simulink model "MtrCtrl_24V"  (R2023b)
settings: Solver=FixedStepDiscrete  StartTime=0.0  StopTime=1  FixedStep=1e-6  RelTol=1e-3
values from neighbouring files (symbols this model uses):
  B = 0.001889    [MtrCtrl_v01.sldd]    (also in PICal.m = 0.001889; PMSM.m = Simulink.Parameter)
  C_LUT_AngleTable_sng_Null = saveVarsMat.C_LUT_AngleTable_sng_Null    [AngleTable.m]    (also in MtrCtrl_v01.sldd = 0.0015339807878856412 0.0030679615757712823 0.00460194236365; PMSM.m; SinLut.m = sinTable(2,:))
  C_LUT_SinTable_sng_Null = saveVarsMat.C_LUT_SinTable_sng_Null    [AngleTable.m]    (also in MtrCtrl_v01.sldd = 0.0015339801862847655 0.0030679567629659761 0.00460192612044; PMSM.m; SinLut.m = sinTable(1,:))
  C_MATH_OneOverSqrtThree_s32n31_Null = 0.57735026918962584    [MtrCtrl_v01.sldd]    (also in PMSM.m = Simulink.Parameter)
  C_MATH_Pi_u32n30_Null = 3.1415926535897931    [MtrCtrl_v01.sldd]    (also in PMSM.m = Simulink.Parameter)
  C_MATH_SqrtThreeOverThree_s32n31_Null = 0.57735026918962573    [MtrCtrl_v01.sldd]    (also in PMSM.m = Simulink.Parameter)
  C_PMSM_CurQKi_u32n31_null = 0.15707963267949    [MtrCtrl_v01.sldd]    (also in PMSM.m = Simulink.Parameter)
  C_PMSM_CurQKp_u32n31_null = 19.949113350295185    [MtrCtrl_v01.sldd]    (also in PMSM.m = Simulink.Parameter)
  C_PMSM_Flux_u32n32_Vs = 0.192    [MtrCtrl_v01.sldd]    (also in PMSM.m = Simulink.Parameter)
  C_PMSM_Ls_pu = 0.398982267005904    [MtrCtrl_v01.sldd]
  C_PMSM_PolePairs_u8_Null = 4.0    [MtrCtrl_v01.sldd]
  Flux = 0.192    [MtrCtrl_v01.sldd]    (also in PICal.m; PMSM.m)
  IBase_A = 2000.0    [MtrCtrl_v01.sldd]    (also in PICal.m = 300; PMSM.m = Simulink.Parameter)
  J = 0.011    [MtrCtrl_v01.sldd]    (also in PICal.m; PMSM.m)
  K_CCM_MRASEna_bool_Flg = 0.0    [MtrCtrl_v01.sldd]
  K_SVM_DefultDuty_s32n31_Null = 0.25    [MtrCtrl_v01.sldd]    (also in PMSM.m = Simulink.Parameter)
  KCCM_VirPosn_flg = 0.0    [MtrCtrl_v01.sldd]    (also in PMSM.m = Simulink.Parameter)
  KCCM_VoltModeEna_Flg = 0.0    [MtrCtrl_v01.sldd]    (also in PMSM.m = Simulink.Parameter)
  Kis = 114583.3333333333    [MtrCtrl_v01.sldd]    (also in PICal.m = 114583.333333; PMSM.m = 114583.333333)
  KSMO_EnaEst_Flg = 0.0    [MtrCtrl_v01.sldd]    (also in PMSM.m = Simulink.Parameter)
  Kt = 1.1520000000000001    [MtrCtrl_v01.sldd]    (also in PICal.m = 1.152; PMSM.m = 1.152)
  Ld = 80e-6    (= 8e-05)    [FluxweakingGen.m]    (also in IEHB_MAPGenerationtest.m = 6.8e-05; MtrCtrl_v01.sldd = 0.000635
                
                    
             ; PICal.m = 0.000635; PMSM.m = Simulink.Parameter)
  LPF_coefg = 0.01    [MtrCtrl_v01.sldd]    (also in PMSM.m = Simulink.Parameter)
  Lq = 80e-6    (= 8e-05)    [FluxweakingGen.m]    (also in IEHB_MAPGenerationtest.m = 6e-05; MtrCtrl_v01.sldd = 0.000685
                
                    
             ; PICal.m = 0.000635; PMSM.m = Simulink.Parameter)
  Ls = 0.000635    [MtrCtrl_v01.sldd]    (also in PICal.m; PMSM.m)
  OneOverUBase_V = 0.0016666666666666668    [MtrCtrl_v01.sldd]    (also in PMSM.m = Simulink.Parameter)
  Pp = 4.0    [MtrCtrl_v01.sldd]    (also in PICal.m = 4; PMSM.m = Simulink.Parameter)
  Rs = 0.03    [FluxweakingGen.m]    (also in MtrCtrl_v01.sldd = 0.05
                
                    
                 ; PICal.m = 0.05; PMSM.m = Simulink.Parameter)
  SecPerRnd = 0.6    [MtrCtrl_v01.sldd]    (also in PMSM.m = Simulink.Parameter)
  sinTable = zeros(2,TableSize)    [SinLut.m]
  SMOGain_V = 323.31615074619043    [MtrCtrl_v01.sldd]    (also in PMSM.m = Simulink.Parameter)
  Ts = 1.0E-6    [MtrCtrl_v01.sldd]    (also in PICal.m = 0.0001; PMSM.m = Simulink.Parameter)
  TsCtrl = 1.0E-6    [MtrCtrl_v01.sldd]
  UBase_V = 600.0    [MtrCtrl_v01.sldd]    (also in PICal.m = 600; PMSM.m = Simulink.Parameter)
  wmBase_rps = 314.15926535897933    [MtrCtrl_v01.sldd]    (also in PICal.m = 314.159265359; PMSM.m = Simulink.Parameter)
undefined symbols (not defined in the file or in its folder): DiscIntNeverNeededParam, Ion, Lithium
libraries: ee_lib x16, spsVoltageMeasurementLib x14, simulink x11, spsSeriesRLCBranchLib x6, spsMosfetLib x6, nesl_utility x6, slpidlib x5, spsCurrentMeasurementLib x4, spsParallelRLCBranchLib x3, simulink_extras x2, spspowerguiLib x2, eePmsmFwController x1
(part 1 of 5)
settings Model: DataDictionary=MtrCtrl_v01.sldd  FPTShortcutValueString='{{},{''BaselineRun'',1,1,1,''BaselineRun'','''',{},''M'','''',''''}}'  PauseTimes=0.0842  NumberOfSteps=100  SnapshotBufferSize=1000  SnapshotInterval=1  Creator=ZhangZhehu  LastModifiedBy=z1486
settings OptimizationCC: DefaultParameterBehavior=Inlined  UseDivisionForNetSlopeComputation=on  GainParamInheritBuiltInType=on  UseFloatMulNetSlope=on  DefaultUnderspecifiedDataType=single  InlineInvariantSignals=on  PassReuseOutputArgsAs=Individual arguments  ZeroExternalMemoryAtStartup=off  ZeroInternalMemoryAtStartup=off  NoFixptDivByZeroProtection=on  EfficientFloat2IntCast=on  LifeSpan=1  OptimizeBlockOrder=speed  DifferentSizesBufferReuse=on  EfficientTunableParamExpr=on
settings DebuggingCC: SignalRangeChecking=warning  ParameterTunabilityLossMsg=error  UnconnectedInputMsg=warning  UnconnectedOutputMsg=warning  UnconnectedLineMsg=warning
settings HardwareCC: ProdBitPerPointer=32  ProdBitPerSizeT=32  ProdBitPerPtrDiffT=32  ProdLargestAtomicFloat=None  ProdWordSize=32  ProdLongLongMode=on  ProdHWDeviceType=Infineon->TriCore
settings ModelReferenceCC: EnableRefExpFcnMdlSchedulingChecks=on
settings SFSimCC: MATLABDynamicMemAlloc=off
settings RTWCC: Description=Embedded Coder  SystemTargetFile=ert.tlc  GenCodeOnly=on  TemplateMakefile=ert_default_tmf  BuildConfiguration=Faster Runs  DLArmComputeVersion=19.05
settings CodeAppCC: ForceParamTrailComments=on  IgnoreCustomStorageClasses=off  OperatorAnnotations=on  SimulinkDataObjDesc=on  SFDataObjDesc=on  CustomSymbolStrGlobalVar=rt$N$M  CustomSymbolStrType=$N$M  CustomSymbolStrFcn=$N$M$F  CustomSymbolStrMacro=$N$M  InsertBlockDesc=on
settings ERTTargetCC: TargetLangStandard=C99 (ISO)  GenerateSampleERTMain=on  IncludeMdlTerminateFcn=off  CombineSignalStateStructs=on  SupportComplex=off  SupportNonInlinedSFcns=on  InlinedParameterPlacement=NonHierarchical  ERTCustomFileTemplate=example_file_process.tlc  ERTFilePackagingFormat=CompactWithDataFile

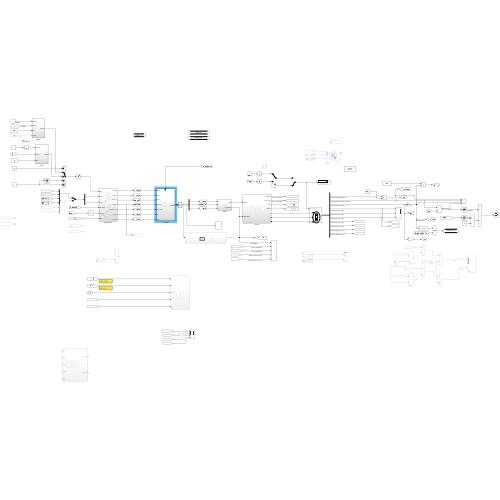
[thumbnail: Simulink's stored preview of the top-level diagram]
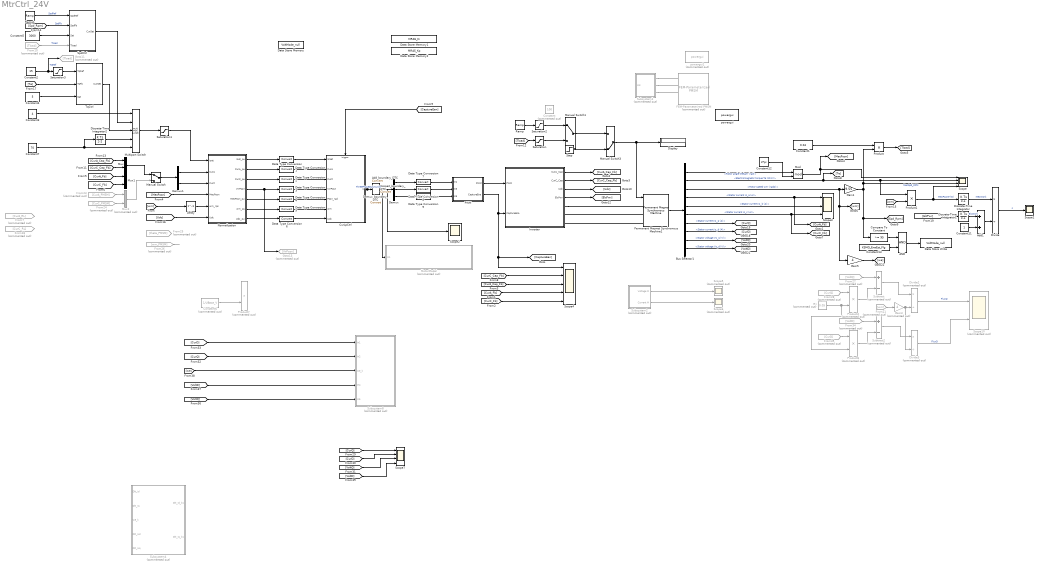
== system MtrCtrl_24V ==
  AND : Logic  AllPortsSameDT=off  OutDataTypeStr=boolean
  Add1 : Sum
  Add_boundary_DTC : DataTypeConversion
  Bus Selector1 : BusSelector  OutputSignals=Rotor angle thetam (rad),Electromagnetic torque Te (N*m),Rotor speed wm (rad/s),Stator current is_a (A),Stator current is_b (A),Stator current is_c (A),Stator current is_q (A),Stator current is_d (A),Stator voltage Vs_q (V),Stator voltage Vs_d (V)
  Compare To Constant : simulink/Logic and Bit Operations/Compare To Constant  relop=>=  const=95  OutDataTypeStr=boolean
  Constant : Constant  Commented=on  Value=100
  Constant1 : Constant  Value=0.04
  Constant11 : Constant
  Constant12 : Constant  Value=2*pi
  Constant13 : Constant  Value=KSMO_EnaEst_Flg
  Constant2 : Constant  Value=15
  Constant3 : Constant  Value=4
  Constant4 : Constant  Value=5
  Constant5 : Constant  Value=3000
  Constant6 : Constant  Commented=on  Value=1/UBase_V
  Constant7 : Constant  Value=70
  CurLpCtrl : Subsystem
      settings: RTWSystemCode=Nonreusable function  RTWFcnNameOpts=Use subsystem name
  Data Store Memory : DataStoreMemory  DataStoreName=VoltMode_null  WriteAfterWriteMsg=warning  ShowAdditionalParam=off
  Data Store Memory1 : DataStoreMemory  DataStoreName=MRAS_Ki  WriteAfterWriteMsg=warning  ShowAdditionalParam=off
  Data Store Memory2 : DataStoreMemory  DataStoreName=MRAS_Kp  WriteAfterWriteMsg=warning  ShowAdditionalParam=off  OutDataTypeStr=fixdt(1,32,27)
  Data Store Write : DataStoreWrite  DataStoreName=VoltMode_null  IndexOptions=Index vector (dialog)  Indices=1  OutputSizes=1
  Data Type Conversion{,1..9} (10 alike) : DataTypeConversion  SaturateOnIntegerOverflow=off  RndMeth=Floor
  Delay : Delay  DelayLength=1
  Demux : Demux  Outputs=3
  Demux1 : Demux  Outputs=2
  Demux_boundary_DTC : DataTypeConversion
  Discrete-Time Integrator : DiscreteIntegrator  SampleTime=-1  ICPrevOutput=DiscIntNeverNeededParam  ICPrevScaledInput=DiscIntNeverNeededParam
  Discrete-Time Integrator1 : DiscreteIntegrator  SampleTime=-1  ICPrevOutput=DiscIntNeverNeededParam  ICPrevScaledInput=DiscIntNeverNeededParam
  Discrete-Time Integrator2 : DiscreteIntegrator  SampleTime=-1  ICPrevOutput=DiscIntNeverNeededParam  ICPrevScaledInput=DiscIntNeverNeededParam
  Display : Display
  Divide : Product  Inputs=*/
  Divide2 : Product  Commented=on  Inputs=*/
  Divide3 : Product  Commented=on  Inputs=*/
  FEM-Parameterized PMSM : ee_lib/Electromechanical/Permanent Magnet/FEM-Parameterized PMSM  Commented=on  parameterization=1  winding_type=ee.enum.statorconnection.wye  iVec=[-2, 0, 2] A  xVec=[0, 20, 40, 60] deg  dfluxdiMatrix=0.0002 * ones(3, 4) Wb/A  dfluxdxMatrix=[0, -.16, .16, 0; 0, -.16, .16, 0; 0, -.16, .16, 0] Wb/rad  calculate_torque_matrix=1  TorqueMatrix=zeros(3, 3, 3, 4) N*m  idVec1=[-200, 0, 200] A  iqVec1=[-200, 0, 200] A  LdMatrix=0.0002 * ones(3, 3) H  LqMatrix=0.0002 * ones(3, 3) H  PmMatrix=0.1 * ones(3, 3) Wb  N=4  interp_method=simscape.enum.interpolation.linear  Rs=0.05 Ohm  Ms=0.00002 H  L0=0.00016 H  loss_param=ee.enum.fem_motor.ironLosses.empirical  losses_oc=[0, 0, 0] W  losses_sc=[0, 0, 0] W  f_losses=60 Hz  Isc_losses=95 A  Inertia=0.01 kg*m^2  lam=0 N*m*s/rad  i_d_specify=off  i_d_priority=None  i_d=0 A  i_d_nominal_specify=off  i_d_nominal_unit=A  i_d_nominal_value=1  i_q_specify=off  i_q_priority=None  i_q=0 A  i_q_nominal_specify=off  i_q_nominal_unit=A  i_q_nominal_value=1  torque_specify=off  torque_priority=None  torque=0 N*m  torque_nominal_specify=off  torque_nominal_unit=N*m  torque_nominal_value=1  angular_velocity_specify=off  angular_velocity_priority=High  angular_velocity=0 rpm  angular_velocity_nominal_specify=off  angular_velocity_nominal_unit=rpm  angular_velocity_nominal_value=1  angular_position_specify=off  angular_position_priority=High  angular_position=0 deg  angular_position_nominal_specify=off  angular_position_nominal_unit=deg  angular_position_nominal_value=1  Tmeas=298.15 K  alpha=3.93e-3 1/K  alpha_flux=-0.001 1/K  stator_thermal_mass=100 J/K  stator_initial_temperatures=[298.15, 298.15, 298.15] K  rotor_thermal_mass=200 J/K  rotor_initial_temperature=298.15 K  Rm_percent_rotor=90  Rd_percent_rotor=30  idVec=[-200, 0, 200] A  iqVec=[-200, 0, 200] A  dfluxAdiaMatrix3D=zeros(3, 3, 4) Wb/A  dfluxAdibMatrix3D=zeros(3, 3, 4) Wb/A  dfluxAdicMatrix3D=zeros(3, 3, 4) Wb/A  dfluxAdxMatrix3D=zeros(3, 3, 4) Wb/rad  TorqueMatrix3D=zeros(3, 3, 4) N*m  iaVec=[-200, 0, 200] A  ibVec=[-200, 0, 200] A  icVec=[-200, 0, 200] A  dfluxAdiaMatrix=zeros(3, 3, 3, 4) Wb/A  dfluxAdibMatrix=zeros(3, 3, 3, 4) Wb/A  dfluxAdicMatrix=zeros(3, 3, 3, 4) Wb/A  dfluxAdxMatrix=zeros(3, 3, 3, 4) Wb/rad  param_dq0=ee.enum.fem_motor.fluxTabulationOption.DQcartesian  winding_type_dq0=ee.enum.statorconnection.wye  expose_neutral_port=ee.enum.fem_motor.exposeNeutralPort.no  nPolePairs=4  parks_type=ee.enum.fem_motor.parksType.QleadsD_AphaseToDaxis  idVec2=[-200, 0, 200] A  iqVec2=[-200, 0, 200] A  magVec2=[0, 100, 200] A  betaVec2=[-180, -90, 0, 90, 180] deg  xVec2=[0, 15, 30, 45, 60, 75, 90] deg  fluxD_dq0=zeros(3, 3, 7) Wb  fluxQ_dq0=zeros(3, 3, 7) Wb  fluxA_dq0=zeros(3, 3, 7) Wb  Torque_dq0=ones(3, 3, 7) N*m  fluxD_IBX=zeros(3, 5, 7) Wb  fluxQ_IBX=zeros(3, 5, 7) Wb  fluxA_IBX=zeros(3, 5, 7) Wb  Torque_IBX=zeros(3, 5, 7) N*m  rotorLossCoeff_k_h_DQ=zeros(3, 3) W/Hz  rotorLossCoeff_k_J_DQ=zeros(3, 3) W/Hz^2  rotorLossCoeff_k_ex_DQ=zeros(3, 3) W/Hz^(3/2)  rotorLossCoeff_k_h_IB=zeros(3, 5) W/Hz  rotorLossCoeff_k_J_IB=zeros(3, 5) W/Hz^2  rotorLossCoeff_k_ex_IB=zeros(3, 5) W/Hz^(3/2)  statorLossCoeff_k_h_DQ=zeros(3, 3) W/Hz  statorLossCoeff_k_J_DQ=zeros(3, 3) W/Hz^2  statorLossCoeff_k_ex_DQ=zeros(3, 3) W/Hz^(3/2)  statorLossCoeff_k_h_IB=zeros(3, 5) W/Hz  statorLossCoeff_k_J_IB=zeros(3, 5) W/Hz^2  statorLossCoeff_k_ex_IB=zeros(3, 5) W/Hz^(3/2)  wVec=[1000, 2000] rpm  rotorLossTable_DQ=zeros(3, 3, 2) W  rotorLossTable_IB=zeros(3, 5, 2) W  statorLossTable_DQ=zeros(3, 3, 2) W  statorLossTable_IB=zeros(3, 5, 2) W  electrical_torque_before_iron_losses_specify=off  electrical_torque_before_iron_losses_priority=None  electrical_torque_before_iron_losses=0 N*m  electrical_torque_before_iron_losses_nominal_specify=off  electrical_torque_before_iron_losses_nominal_unit=N*m  electrical_torque_before_iron_losses_nominal_value=1  Qrotor_specify=off  Qrotor_priority=None  Qrotor=0 J/s  Qrotor_nominal_specify=off  Qrotor_nominal_unit=J/s  Qrotor_nominal_value=1  Qstator_specify=off  Qstator_priority=None  Qstator=0 J/s  Qstator_nominal_specify=off  Qstator_nominal_unit=J/s  Qstator_nominal_value=1
      settings: InternalSimscapePortConfiguration="{\"Bottom\":[],\"Left\":[{\"id\":\"a\",\"label\":\"a\",\"type\":\"foundation.electrical.electrical\"},{\"id\":\"b\",\"label\":\"b\",\"type\":\"foundation.electrical.electrical\"},{\"id\":\"c\",\"label\":\"c\",\"type\":\"foundation.electrical.electrical\"},{\"id\":\"n\",\"label\":\"n\",\"type\":\"foundation.electrical.electrical\"}],\"Right\":[{\"id\":\"R\",\"label\":\"R\",\"type\":\"foundation.mechanical.rotational.rotational\"},{\"id\":\"C\",\"label\":\"C\",\"type\":\"foundation.mechanical.rotational.rotational\"}],\"Top\":[]}"
  From10 : From  Commented=on  GotoTag=Tload
  From18 : From  Commented=on  GotoTag=CurC_RL
  From21 : From  Commented=on  GotoTag=wm
  From23 : From  Commented=on  GotoTag=CurA_PMSM
  From24 : From  Commented=on  GotoTag=CurC_PMSM
  From25 : From  Commented=on  GotoTag=theta_PMSM
  From26 : From  Commented=on  GotoTag=wm_PMSM
  From27 : From  Commented=on  GotoTag=VoltQ
  From28 : From  Commented=on  GotoTag=CurQ
  From34 : From  Commented=on  GotoTag=VoltD
  From35 : From  Commented=on  GotoTag=CurD
  From7 : From  Commented=on  GotoTag=CurA_RL
  Gain1 : Gain  Gain=9.55
  Gain3 : Gain  Commented=on  Gain=4
  Gain5 : Gain  Gain=4
  Goto11 : Goto  Commented=on  GotoTag=Tload
  Goto13 : Goto  Commented=on  GotoTag=VirPosn
  Inverter : Subsystem
  Manual Switch : ManualSwitch
  Manual Switch1 : ManualSwitch
  Manual Switch3 : ManualSwitch  CurrentSetting=0
  Mod : Math  Operator=mod
  MotorModel : Subsystem  Commented=on
  Multiport Switch : MultiPortSwitch  Inputs=4  SaturateOnIntegerOverflow=off  InputSameDT=off
  Mux : Mux  Inputs=2
  Mux1 : Mux  Inputs=2
  Mux2 : Mux  Commented=on  Inputs=2
  Normalization : Subsystem
  PWM : Subsystem
  Permanent Magnet Synchronous Machine1 : spsPermanentMagnetSynchronousMachineLib/Permanent Magnet Synchronous Machine  NbPhases=3  FluxDistribution=Sinusoidal  RotorType=Round  MechanicalLoad=Speed w  PresetModel=No  ShowDetailedParameters=on  MeasurementBus=off  Resistance=0.05  Inductance=6.5e-5  dqInductances=[8.5e-3,8.5e-3]  La=0.000635  MachineConstant=Flux linkage established by magnets (V.s)  Flux=0.192  VoltageCst=139.2998  TorqueCst=1.152  Flat=120  Mechanical=[0.011 0.001889 4 0]  PolePairs=4  InitialConditions=[0,0, 0,0]  InitialConditions5ph=[0 0 0 0 0 0]  RefAngle=Aligned with phase A axis (original Park)  IterativeDiscreteModel=Trapezoidal non iterative  TsBlock=-1  TsPowergui=0
  Product : Product
  Product1 : Product
  Product2 : Product  Commented=on
  Product4 : Product  Commented=on
  Product8 : Product  Commented=on
  Ramp : simulink/Sources/Ramp  slope=30  start=0  InitialOutput=0
  Ramp1 : simulink/Sources/Ramp  slope=2000  start=0  InitialOutput=0
  Rs : Constant  Commented=on  Value=0.05
  Saturation : Saturate  UpperLimit=200  LowerLimit=-5
  Saturation1 : Saturate  UpperLimit=220
  Saturation2 : Saturate  UpperLimit=30
  Saturation3 : Saturate  UpperLimit=11
  Scope : Scope  NumInputPorts=4
  Scope1 : Scope
  Scope10 : Scope  Commented=on  NumInputPorts=2
  Scope2 : Scope
  Scope2_boundary_DTC : DataTypeConversion
  Scope3 : Scope  NumInputPorts=3
  Scope4 : Scope  NumInputPorts=5
  Scope5 : Scope  Commented=on
  Scope6 : Scope  Commented=on
  Scope7 : Scope  NumInputPorts=4
  SpdCtrl : Subsystem
  Step : Step  Time=0.01  After=100  SampleTime=0
  Subsystem1 : Subsystem  Commented=on
  Subsystem2 : Subsystem  Commented=on
  Subsystem4 : Subsystem  Commented=on
  Subsystem8 : Subsystem  Commented=on
  Subtract : Sum  Commented=on  Inputs=+-
  Subtract2 : Sum  Commented=on  Inputs=+-
  TqCtrl : Subsystem
  powergui : spspowerguiLib/powergui  Priority=1  SimulationMode=Discrete  SampleTime=1e-6  frequency=60  Iterations=50  frequencyindice=0  Pbase=100e6  ErrMax=1e-4  UnitsV=kV  UnitsW=MW  buscounter=0  FunctionMessages=off  echomessages=off  EnableUseOfTLC=off  CurrentSourceSwitches=off  DisableSnubberDevices=off  DisableRonSwitches=off  DisableVfSwitches=off  DisplayEquations=off  AutomaticDiscreteSolvers=off  SolverType=Tustin/Backward Euler (TBE)  Interpol=off  ExternalGateDelay=off  methode=off  Ts=100  x0status=blocks  SPID=on  SwTol=0  HookPort=off  NonlinearTolerance=1e-4  nMaxIteration=100  ContinueOnMaxIteration=off  RestoreLinks=warning  ResistiveCurrentMeasurement=off  Frange=[0:2:500]  Ylog=off  Xlog=on  ShowGrid=off  save=off  variable=ZData  structure=0  ZoomFFT=off  StartTime=0.0  cycles=1  DisplayStyle=1  fundamental=60  FreqAxis=off  MaxFrequency=1000  frequencyindicesteady=1  RmsSteady=1  display=off
  powergui1 : spspowerguiLib/powergui  Priority=1  Commented=on  SimulationMode=Continuous  SampleTime=50e-6  frequency=60  Iterations=50  frequencyindice=60  Pbase=100e6  ErrMax=1e-4  UnitsV=kV  UnitsW=MW  buscounter=0  FunctionMessages=off  echomessages=off  EnableUseOfTLC=off  CurrentSourceSwitches=off  DisableSnubberDevices=off  DisableRonSwitches=off  DisableVfSwitches=off  DisplayEquations=off  AutomaticDiscreteSolvers=off  SolverType=Tustin/Backward Euler (TBE)  Interpol=off  ExternalGateDelay=off  methode=off  Ts=100  x0status=blocks  SPID=on  SwTol=0  HookPort=off  NonlinearTolerance=1e-4  nMaxIteration=100  ContinueOnMaxIteration=off  RestoreLinks=warning  ResistiveCurrentMeasurement=off  Frange=[0:2:500]  Ylog=off  Xlog=on  ShowGrid=off  save=off  variable=ZData  structure=0  ZoomFFT=off  StartTime=0.0  cycles=1  DisplayStyle=1  fundamental=60  FreqAxis=off  MaxFrequency=1000  frequencyindicesteady=1  RmsSteady=1  display=off
  wires:
  Ramp/1 -> Saturation2/1
  Bus Selector1/4 -> Scope3/1, [CurA_Fb]  "<Stator current is_a (A)>"
  Bus Selector1/2 -> [Te], Scope/2, Product1/1  "<Electromagnetic torque Te (N*m)>"
  Mod/1 -> [MecPosn], Scope/1
  Permanent Magnet Synchronous Machine1/1 -> Bus Selector1/1
  Bus Selector1/6 -> Scope3/3, [CurC_Fb]  "<Stator current is_c (A)>"
  Bus Selector1/3 -> Gain5/1, [wm], Gain1/1  "<Rotor speed wm (rad/s)>"
  Gain1/1 -> Compare To Constant/1, [Spd_Rpm], Product/2, Scope/3  "MecSpd_RPM"
  Constant1/1 -> Product/1
  Product/1 -> [Tload]
  PWM/1(PWM) -> Inverter/1(PWM)
  Demux/3 -> Data Type Conversion9/1
  Demux/1 -> Data Type Conversion7/1
  Demux/2 -> Data Type Conversion8/1
  PWM/2(CaptureEna) -> [CaptureEan], Scope4/1, Inverter/2(CaptureEna)
  From26/1 -> ?
  Inverter/2(CurC_Cap) -> [CurC_Cap_Fb]
  Inverter/1(CurA_Cap) -> [CurA_Cap_Fb]
  Bus Selector1/5 -> Scope3/2  "<Stator current is_b (A)>"
  [CurA_Fb] -> Scope4/4
  [CurC_Fb] -> Scope4/5
  [CurC_Cap_Fb] -> Scope4/2
  [CurA_Cap_Fb] -> Scope4/3
  [CaptureEan] -> CurLpCtrl/Trigger
  [wm] -> Product1/2
  Inverter/3(Udc) -> [Udc]
  Ramp1/1 -> SpdCtrl/1(SpdRef)  "SpdRef"
  [Spd_Rpm] -> SpdCtrl/2(SpdFb)  "SpdFb"
  Constant5/1 -> SpdCtrl/3(Sat)
  From10/1 -> SpdCtrl/4(Tload)  "Tload"
  SpdCtrl/1(CurSet) -> Multiport Switch/2
  TqCtrl/1(CurSet) -> Multiport Switch/3
  [Te] -> TqCtrl/2(TqFb)
  Constant2/1 -> Goto11/1, Saturation3/1  "TqRef"
  Constant4/1 -> TqCtrl/3(Sat)
  [Tload] -> Saturation/1
  Saturation/1 -> Manual Switch1/2
  Saturation2/1 -> Manual Switch1/1
  Manual Switch/1 -> Demux1/1
  Mux2/1 -> Manual Switch/2
  [CurC_Cap_Fb] -> Mux/2
  [CurA_Cap_Fb] -> Mux/1
  Mux/1 -> Manual Switch/1
  [CurC_Fb] -> Mux1/2
  [CurA_Fb] -> Mux1/1
  Manual Switch3/1 -> Display/1, Permanent Magnet Synchronous Machine1/1
  Manual Switch1/1 -> Manual Switch3/1
  Product1/1 -> Discrete-Time Integrator/1, Scope/4  "MecPower(W)"
  Saturation3/1 -> TqCtrl/1(TqRef)
  Inverter/4(ElcPwr) -> [ElcPwr]
  Discrete-Time Integrator/1 -> Divide/1  "MecWork"
  [ElcPwr] -> Discrete-Time Integrator1/1
  Discrete-Time Integrator1/1 -> Add1/1  "ElcWork"
  Divide/1 -> Scope1/1  "n"
  Step/1 -> Manual Switch3/2
  Constant6/1 -> Product2/2
  Multiport Switch/1 -> Saturation1/1
  Demux1/1 -> Normalization/2(CurA)
  Demux1/2 -> Normalization/3(CurC)
  [MecPosn] -> Normalization/4(MecPosn)
  Delay/1 -> Normalization/5(wm_rps)
  [Udc] -> Normalization/6(Udc)
  Constant7/1 -> Discrete-Time Integrator2/1, Multiport Switch/5
  Constant3/1 -> Multiport Switch/1
  Discrete-Time Integrator2/1 -> Multiport Switch/4
  Saturation1/1 -> Normalization/1(Iset)
  Subsystem2/1(Voltage M) -> Scope5/1
  Subsystem2/2(Current M) -> Scope6/1
  From23/1 -> Mux2/1
  From24/1 -> Mux2/2
  Add1/1 -> Divide/2
  Constant11/1 -> Add1/2
  [wm] -> Delay/1
  Compare To Constant/1 -> AND/1
  Normalization/1(Iset_pu) -> Data Type Conversion/1
  Normalization/2(CurA_pu) -> Data Type Conversion1/1
  Normalization/3(CurC_pu) -> Data Type Conversion2/1
  Normalization/4(VirPosn) -> Data Type Conversion3/1, Goto13/1
  Normalization/5(MecPosn_pu) -> Data Type Conversion4/1
  Normalization/6(wm_pu) -> Data Type Conversion5/1
  Normalization/7(Udc_pu) -> Data Type Conversion6/1
  CurLpCtrl/1(S) -> Add_boundary_DTC/1, Demux_boundary_DTC/1, Scope2_boundary_DTC/1  "ThreePhaseDutyCycle"
  Data Type Conversion/1 -> CurLpCtrl/1(IsSet)
  Data Type Conversion1/1 -> CurLpCtrl/2(CurA)
  Data Type Conversion2/1 -> CurLpCtrl/3(CurC)
  Data Type Conversion3/1 -> CurLpCtrl/4(VirPosn)
  Data Type Conversion4/1 -> CurLpCtrl/5(Posn_rad)
  Data Type Conversion5/1 -> CurLpCtrl/6(wm)
  Data Type Conversion6/1 -> CurLpCtrl/7(Udc)
  Data Type Conversion7/1 -> PWM/1(In1)
  Data Type Conversion8/1 -> PWM/2(In3)
  Data Type Conversion9/1 -> PWM/3(In5)
  Demux_boundary_DTC/1 -> Demux/1
  Scope2_boundary_DTC/1 -> Scope2/1
  Bus Selector1/1 -> Mod/1  "<Rotor angle thetam (rad)>"
  Constant12/1 -> Mod/2
  AND/1 -> Data Store Write/1
  Constant13/1 -> AND/2
  Bus Selector1/7 -> [CurQ]  "<Stator current is_q (A)>"
  Bus Selector1/8 -> [CurD]  "<Stator current is_d (A)>"
  Bus Selector1/9 -> [VoltQ]  "<Stator voltage Vs_q (V)>"
  Bus Selector1/10 -> [VoltD]  "<Stator voltage Vs_d (V)>"
  Product4/1 -> Subtract/2
  Subtract/1 -> Divide2/1
  From21/1 -> Gain3/1
  Divide2/1 -> Scope10/1  "FluxQ"
  Gain3/1 -> Divide3/2, Divide2/2
  From27/1 -> Subtract/1
  From28/1 -> Product4/1
  From35/1 -> Product8/1
  From34/1 -> Subtract2/1
  Subtract2/1 -> Divide3/1
  Product8/1 -> Subtract2/2
  Rs/1 -> Product8/2, Product4/2
  Divide3/1 -> Scope10/2  "FluxD"
  Gain5/1 -> [we]
  Add_boundary_DTC/1 -> MotorModel/1(In1)
  [CurD] -> Subsystem8/1(In1)
  [CurQ] -> Subsystem8/2(In2)
  [we] -> Subsystem8/3(we_k)
  [VoltD] -> Subsystem8/4(In4)
  [VoltQ] -> Subsystem8/5(In5)
  [CurD] -> Scope7/2
  [VoltD] -> Scope7/4
  [CurQ] -> Scope7/1
  [VoltQ] -> Scope7/3
  connections:
  Inverter/RConn1 -- Permanent Magnet Synchronous Machine1/LConn1
  Permanent Magnet Synchronous Machine1/LConn2 -- Inverter/RConn2
  Permanent Magnet Synchronous Machine1/LConn3 -- Inverter/RConn3
  Subsystem1/RConn2 -- FEM-Parameterized PMSM/LConn2
  Subsystem1/RConn3 -- FEM-Parameterized PMSM/LConn3
  Subsystem1/RConn1 -- FEM-Parameterized PMSM/LConn1

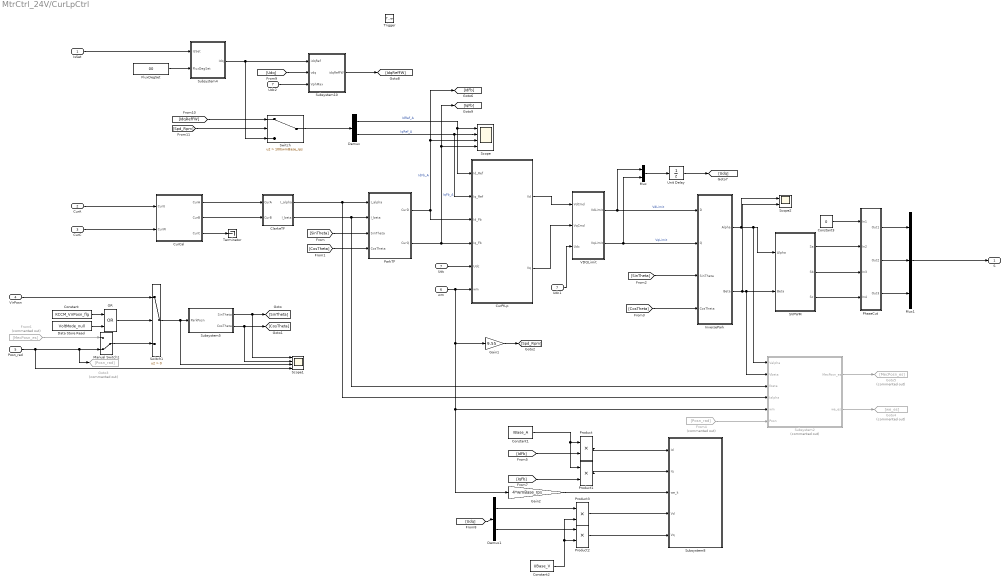
== system MtrCtrl_24V/CurLpCtrl ==
  IsSet : Inport  OutDataTypeStr=fixdt(1,32,31)
  CurA : Inport  Port=2  OutDataTypeStr=fixdt(1,32,31)
  CurC : Inport  Port=3  OutDataTypeStr=fixdt(1,32,31)
  VirPosn : Inport  Port=4  OutDataTypeStr=fixdt(1,32,28)
  Posn_rad : Inport  Port=5  OutDataTypeStr=fixdt(1,32,28)
  wm : Inport  Port=6  OutDataTypeStr=fixdt(1,32,31)
  Udc : Inport  Port=7  OutDataTypeStr=fixdt(0,32,32)
  Trigger : TriggerPort  VariantControl=(inherit)  PortDimensions=1
  ClarkeTF : Subsystem
  Constant : Constant  Value=KCCM_VirPosn_flg
  Constant1 : Constant  Value=IBase_A
  Constant2 : Constant  Value=UBase_V
  Constant3 : Constant  Value=0  OutDataTypeStr=fixdt(1,32,4)
  CurCal : Subsystem
  CurPILp : Subsystem
  Data Store Read : DataStoreRead  DataStoreName=VoltMode_null  IndexOptions=Index vector (dialog)  Indices=1  OutputSizes=1
  Demux : Demux  Outputs=2
  Demux1 : Demux  Outputs=2
  FluxDegSet : Constant  Value=00  OutDataTypeStr=fixdt(1,32,4)
  From4 : From  Commented=on  GotoTag=Posn_rad
  From6 : From  Commented=on  GotoTag=MecPosn_es
  Gain1 : Gain  Gain=9.55  OutDataTypeStr=fixdt(0,32,30)
  Gain2 : Gain  Gain=4*wmBase_rps  OutDataTypeStr=single
  Goto3 : Goto  Commented=on  GotoTag=Posn_rad
  Goto4 : Goto  Commented=on  GotoTag=we_es
  Goto5 : Goto  Commented=on  GotoTag=MecPosn_es
  InversePark : Subsystem
  Manual Switch1 : ManualSwitch  CurrentSetting=0
  Mux : Mux  Inputs=2
  Mux1 : Mux  Inputs=3
  OR : Logic  Operator=OR  AllPortsSameDT=off  OutDataTypeStr=boolean
  ParkTF : Subsystem
  PhaseCut : Subsystem
  Product{,1..3} (4 alike) : Product  OutDataTypeStr=single
  SVPWM : Subsystem
  Scope : Scope  NumInputPorts=4
  Scope1 : Scope  NumInputPorts=4
  Scope2 : Scope  NumInputPorts=2
  Subsystem10 : Subsystem
  Subsystem2 : Subsystem  Commented=on
  Subsystem4 : Subsystem
  Subsystem5 : Subsystem
  Subsystem8 : Subsystem
  Switch : Switch  Criteria=u2 > Threshold  Threshold=100/wmBase_rps  OutDataTypeStr=fixdt(1,32,31)  SaturateOnIntegerOverflow=off  InputSameDT=off
  Switch1 : Switch  Criteria=u2 > Threshold  OutDataTypeStr=fixdt(1,32,28)  SaturateOnIntegerOverflow=off  InputSameDT=off
  Terminator : Terminator
  Udc1 : InportShadow  Port=7  OutDataTypeStr=fixdt(0,32,32)
  Udc2 : InportShadow  Port=7  OutDataTypeStr=fixdt(0,32,32)
  Unit Delay : UnitDelay  SampleTime=-1  HasFrameUpgradeWarning=on
  VDQLimit : Subsystem
  S : Outport
  wires:
  Subsystem10/1(idqRefFW) -> [IdqRefFW]
  Demux/1 -> CurPILp/1(Id_Ref), Scope/1  "IdRef_A"
  [IdqRefFW] -> Switch/1
  [SinTheta] -> InversePark/3(SinTheta)
  Mux/1 -> Unit Delay/1
  ParkTF/2(CurQ) -> [IqFb], Scope/4, CurPILp/4(Iq_Fb)  "IqFb_A"
  VirPosn/1 -> Switch1/1
  CurPILp/1(Vd) -> VDQLimit/1(VdCmd)
  CurA/1 -> CurCal/1(CurU)
  CurPILp/2(Vq) -> VDQLimit/2(VqCmd)
  Switch/1 -> Demux/1
  Subsystem5/1(SinTheta) -> Scope1/1, [SinTheta]
  [Spd_Rpm] -> Switch/2
  Subsystem5/2(CosTheta) -> Scope1/2, [CosTheta]
  ParkTF/1(CurD) -> [IdFb], Scope/3, CurPILp/3(Id_Fb)  "IdFb_A"
  [Udq] -> Subsystem10/2(vdq)
  CurCal/1(CurA) -> ClarkeTF/1(CurA)
  ClarkeTF/2(I_beta) -> Subsystem2/3(Ibeta), ParkTF/2(I_beta)
  ClarkeTF/1(I_alpha) -> Subsystem2/4(Ialpha), ParkTF/1(I_alpha)
  CurC/1 -> CurCal/2(CurW)
  FluxDegSet/1 -> Subsystem4/2(FluxDegSet)
  [CosTheta] -> ParkTF/4(CosTheta)
  Mux1/1 -> S/1
  [CosTheta] -> InversePark/4(CosTheta)
  [SinTheta] -> ParkTF/3(SinTheta)
  InversePark/2(Beta) -> Scope2/2, Subsystem2/2(Vbeta), SVPWM/2(Beta)
  Demux/2 -> CurPILp/2(Iq_Ref), Scope/2  "IqRef_A"
  CurCal/2(CurB) -> ClarkeTF/2(CurB)
  Manual Switch1/1 -> Switch1/3
  wm/1 -> CurPILp/6(wm), Gain2/1, Subsystem2/5(wm), Gain1/1
  Gain1/1 -> [Spd_Rpm]
  Subsystem4/1(Idq) -> Switch/3, Subsystem10/1(idqRef)
  VDQLimit/1(VdLimit) -> Mux/1, InversePark/1(D)  "VdLimit"
  VDQLimit/2(VqLimit) -> Mux/2, InversePark/2(Q)  "VqLimit"
  Udc/1 -> CurPILp/5(Udc)
  Udc2/1 -> Subsystem10/3(VphMax)
  Unit Delay/1 -> [Udq]
  Constant3/1 -> PhaseCut/1(In1)
  SVPWM/1(Sa) -> PhaseCut/2(In2)
  SVPWM/2(Sb) -> PhaseCut/3(In3)
  SVPWM/3(Sc) -> PhaseCut/4(In4)
  PhaseCut/1(Out1) -> Mux1/1
  PhaseCut/2(Out2) -> Mux1/2
  PhaseCut/3(Out3) -> Mux1/3
  IsSet/1 -> Subsystem4/1(IsSet)
  Udc1/1 -> VDQLimit/3(Udc)
  InversePark/1(Alpha) -> Scope2/1, Subsystem2/1(Valpha), SVPWM/1(Alpha)
  From4/1 -> Subsystem2/6(Posn)
  Subsystem2/2(we_es) -> Goto4/1
  Subsystem2/1(MecPosn_es) -> Goto5/1
  Posn_rad/1 -> Scope1/4, Manual Switch1/2, Goto3/1
  From6/1 -> Manual Switch1/1
  Switch1/1 -> Scope1/3, Subsystem5/1(ParkPosn)
  Constant/1 -> OR/1
  Data Store Read/1 -> OR/2
  OR/1 -> Switch1/2
  CurCal/3(CurC) -> Terminator/1
  [IqFb] -> Product1/2
  [IdFb] -> Product/2
  Gain2/1 -> Subsystem8/3(we_k)
  [Udq] -> Demux1/1
  Demux1/1 -> Product3/1
  Demux1/2 -> Product2/1
  Constant1/1 -> Product/1, Product1/1
  Product/1 -> Subsystem8/1(Id)
  Product1/1 -> Subsystem8/2(Iq)
  Product3/1 -> Subsystem8/4(Vd)
  Product2/1 -> Subsystem8/5(Vq)
  Constant2/1 -> Product3/2, Product2/2

== system MtrCtrl_24V/Inverter ==
  PWM : Inport
  CaptureEna : Inport  Port=2
  Battery : spsBatteryLib/Battery  Commented=on  BatType=Lithium-Ion  ShowTempParam=off  ThermalPreset="12.8V  40Ah  (LiFeMgPO4)"  ShowAgeParam=off  NomV=13.5  NomQ=40  SOC=100  Batt_Tr=30  PresetModel=off  MaxQ=40  MinV=10.5  FullV=14.5  Dis_rate=20  R=0.015  Normal_OP=30.14  expZone="[14.1          0.5]"  current=[6.5 13 32.5]  Units=Time  Tci=20  NomT=20  T2=0  MaxQ2=36  FullV2=13  Normal_OP2=11.7  expZone2="[12.67            4]"  Rca=0.6411  ti=4880  Dp=0  Neq0=0  Tsim=1e6  Ta1=25  Qeol=5.4*0.9  Reol=0.013333*1.2  Char_age=[2.3478, 3]  Dis_age=[2.3478, 10]  N1=1500  N2=10500  N3=1000  N4=1400  Ta2=45  N5=950
  Bus Selector : BusSelector  Commented=on  OutputSignals=Current (A),Voltage (V)
  Current Measurement : spsCurrentMeasurementLib/Current Measurement  PhasorSimulation=off  OutputType=Complex  PSBequivalent=0
  DC Voltage Source : spsDCVoltageSourceLib/DC Voltage Source  Amplitude=570  Measurements=Voltage
  Discrete-Time Integrator : DiscreteIntegrator  Commented=on  SampleTime=-1  ICPrevOutput=DiscIntNeverNeededParam  ICPrevScaledInput=DiscIntNeverNeededParam
  Product : Product  Commented=on
  Product1 : Product
  Scope : Scope  Commented=on  NumInputPorts=3
  Scope1 : Scope  Commented=on
  Scope2 : Scope  NumInputPorts=3
  Series RLC Branch : spsSeriesRLCBranchLib/Series RLC Branch  LConnTagsString=__new0  RConnTagsString=__new0  BranchType=C  Resistance=1  Inductance=1e-3  SetiL0=off  InitialCurrent=0  Capacitance=1e-3  Setx0=off  InitialVoltage=0  Measurements=None
  Series RLC Branch1 : spsSeriesRLCBranchLib/Series RLC Branch  LConnTagsString=__new0  RConnTagsString=__new0  BranchType=R  Resistance=0.0005  Inductance=1e-3  SetiL0=off  InitialCurrent=0  Capacitance=1e-3  Setx0=off  InitialVoltage=0  Measurements=None
  Subsystem : Subsystem
  Universal Bridge : spsUniversalBridgeLib/Universal Bridge  Commented=on  Arms=3  SnubberResistance=1e5  SnubberCapacitance=inf  Device=IGBT / Diodes  Ron=1e-3  Lon=0  ForwardVoltages="[  0  0  ]"  ForwardVoltage=0  GTOparameters=[ 10e-6 , 20e-6 ]  IGBTparameters=[ 1e-6 , 2e-6 ]  Measurements=None  Measurements_2=None  converterType=Rectifier
  Voltage Measurement : spsVoltageMeasurementLib/Voltage Measurement  PhasorSimulation=off  OutputType=Complex  PSBequivalent=0
  A : PMIOPort  Side=Right
  B : PMIOPort  Port=2  Side=Right
  C : PMIOPort  Port=3  Side=Right
  CurA_Cap : Outport
  CurC_Cap : Outport  Port=2
  Udc : Outport  Port=3
  ElcPwr : Outport  Port=4
  wires:
  PWM/1 -> Subsystem/1(In1)
  CaptureEna/1 -> Subsystem/2(CaptureEna)
  Subsystem/1(CurA_Cap) -> CurA_Cap/1
  Subsystem/2(CurC_Cap) -> CurC_Cap/1
  Discrete-Time Integrator/1 -> Scope1/1
  Bus Selector/2 -> Product/2, Scope/2  "<Voltage (V)>"
  Bus Selector/1 -> Product/1, Scope/1  "<Current (A)>"
  Product/1 -> Scope/3, Discrete-Time Integrator/1  "Power(W)"
  Battery/1 -> Bus Selector/1
  Voltage Measurement/1 -> Product1/1, Scope2/2, Udc/1  "Udc"
  Current Measurement/1 -> Product1/2, Scope2/3  "Is"
  Product1/1 -> ElcPwr/1, Scope2/1  "ElcPower_W"
  connections:
  Voltage Measurement/LConn1 -- DC Voltage Source/RConn1 -- Current Measurement/LConn1
  DC Voltage Source/LConn1 -- Series RLC Branch/RConn1 -- Subsystem/LConn2 -- Voltage Measurement/LConn2
  A/RConn1 -- Subsystem/RConn1
  B/RConn1 -- Subsystem/RConn2
  C/RConn1 -- Subsystem/RConn3
  Series RLC Branch/LConn1 -- Series RLC Branch1/LConn1 -- Subsystem/LConn1
  Current Measurement/RConn1 -- Series RLC Branch1/RConn1

== system MtrCtrl_24V/MotorModel ==
  note: 经过三角载波调制后，再乘这个矩阵，再乘以1/3与Udc，
      | 即可得到真实的“相电压”。(注意，这里的“相电压”其实不是
      | 相电压，应该是端电压，即电机端到地的电压，相电压应
      | 该是正弦)为什么乘以这个矩阵暂时不知道，但结果是对的。
      | 关于结果可查看表“开关状态与相电压和线电压的对应关系”。
  In1 : Inport
  Add : Sum
  Bus Selector : BusSelector  OutputSignals=CurA,CurB,CurC
  Bus Selector2 : BusSelector  OutputSignals=Id,Iq
  Bus Selector3 : BusSelector  OutputSignals=CurA,CurC
  Constant10 : Constant  Value=0.25
  Constant8 : Constant  Value=[2 -1 -1;-1 2 -1;-1 -1 2]
  Constant9 : Constant  Value=10
  Demux2 : Demux  Outputs=3
  Display1 : Display
  Divide1 : Product  Inputs=**
  Gain : Gain  Gain=1/3
  Gain2 : Gain  Gain=-1
  Product3 : Product  Multiplication=Matrix(*)  RndMeth=Zero
  Scope7 : Scope  NumInputPorts=4
  Scope8 : Scope  NumInputPorts=3
  Scope9 : Scope  NumInputPorts=2
  Subsystem : Subsystem  mask{Ld=Ls, Lq=Ls, Rs=Rs, Flux=Flux, J=J, B=B, MaxSpd=10000, Pp=4, PosnSelector=0}
      mask prompts: Rs "Phase Resisitor"; Flux "Flux Linkage"; J "Inertia"; B "Viscous damping"; MaxSpd "Max speed set"; Pp "Pole pairs"; PosnSelector "VirPosnEna"
      mask Display: disp("PMSM_111Nm_3000RPM_560V-129Nm")
  wires:
  Product3/1 -> Divide1/1
  Subsystem/5(CurMaesure) -> Bus Selector/1, Bus Selector3/1, Bus Selector2/1
  Constant10/1 -> Add/2
  Gain/1 -> Divide1/2
  Subsystem/2(wm) -> [wm_PMSM], Scope7/2
  Bus Selector/3 -> Scope8/3  "<CurC>"
  Bus Selector/1 -> Scope8/1  "<CurA>"
  Add/1 -> Gain2/1
  Subsystem/1(Te) -> Scope7/1
  [VirPosn] -> Subsystem/5(Theta_In)
  Constant8/1 -> Product3/1, Display1/1
  Bus Selector2/2 -> Scope9/2  "<Iq>"
  Constant9/1 -> Subsystem/1(TLoad)
  Demux2/3 -> Subsystem/4(Vc)
  Bus Selector2/1 -> Scope9/1  "<Id>"
  Subsystem/3(Speed_rpm) -> Scope7/3
  Bus Selector3/1 -> [CurA_PMSM]  "<CurA>"
  Subsystem/4(theta) -> [theta_PMSM], Scope7/4
  Bus Selector3/2 -> [CurC_PMSM]  "<CurC>"
  Demux2/2 -> Subsystem/3(Vb)
  Divide1/1 -> Demux2/1
  Demux2/1 -> Subsystem/2(Va)
  [Udc] -> Gain/1
  Bus Selector/2 -> Scope8/2  "<CurB>"
  Gain2/1 -> Product3/2
  In1/1 -> Add/1

== system MtrCtrl_24V/Normalization ==
  Iset : Inport
  CurA : Inport  Port=2
  CurC : Inport  Port=3
  MecPosn : Inport  Port=4
  wm_rps : Inport  Port=5
  Udc : Inport  Port=6
  Constant : Constant
  Constant1 : Constant  Value=1/IBase_A
  Constant10 : Constant  Value=1/wmBase_rps
  Constant3 : Constant  Value=1/UBase_V
  Product{3..8} (6 alike) : Product
  Repeating Sequence : simulink/Sources/Repeating Sequence  rep_seq_t=[0 SecPerRnd]  rep_seq_y=[0 2*pi]
  Scope : Scope  NumInputPorts=2
  Scope1 : Scope
  Iset_pu : Outport
  CurA_pu : Outport  Port=2
  CurC_pu : Outport  Port=3
  VirPosn : Outport  Port=4
  MecPosn_pu : Outport  Port=5
  wm_pu : Outport  Port=6
  Udc_pu : Outport  Port=7
  wires:
  Product6/1 -> Iset_pu/1
  Product4/1 -> wm_pu/1
  Constant1/1 -> Product6/2, Product5/2, Product7/2
  Product3/1 -> Udc_pu/1
  Constant10/1 -> Product4/2
  Constant3/1 -> Product3/2
  MecPosn/1 -> Product8/1
  CurC/1 -> Product7/1
  Product5/1 -> Scope/1, CurA_pu/1
  Product7/1 -> Scope/2, CurC_pu/1
  CurA/1 -> Product5/1
  Udc/1 -> Product3/1
  Product8/1 -> Scope1/1, MecPosn_pu/1
  wm_rps/1 -> Product4/1
  Constant/1 -> Product8/2
  Repeating Sequence/1 -> VirPosn/1
  Iset/1 -> Product6/1

== system MtrCtrl_24V/PWM ==
  In1 : Inport
  In3 : Inport  Port=2
  In5 : Inport  Port=3
  Compare To Constant : simulink/Logic and Bit Operations/Compare To Constant  relop=<=  const=0.003  OutDataTypeStr=boolean
  Gain : Gain  Gain=0.3
  Gain1 : Gain  Gain=0.6
  Mux : Mux  Inputs=6
  NOT : Logic  Operator=NOT  AllPortsSameDT=off  OutDataTypeStr=boolean
  NOT1 : Logic  Operator=NOT  AllPortsSameDT=off  OutDataTypeStr=boolean
  NOT2 : Logic  Operator=NOT  AllPortsSameDT=off  OutDataTypeStr=boolean
  Relational Operator : RelationalOperator  Operator=<=  OutDataTypeStr=boolean  RndMeth=Simplest  InputSameDT=off
  Relational Operator1 : RelationalOperator  Operator=<=  OutDataTypeStr=boolean  RndMeth=Simplest  InputSameDT=off
  Relational Operator2 : RelationalOperator  Operator=<=  OutDataTypeStr=boolean  RndMeth=Simplest  InputSameDT=off
  Repeating Sequence : simulink/Sources/Repeating Sequence  rep_seq_t=[0 Ts*100/2 Ts*100]  rep_seq_y=[0 0.5 0]
  Scope : Scope  NumInputPorts=4
  Scope2 : Scope  NumInputPorts=6
  PWM : Outport
  CaptureEna : Outport  Port=2
  wires:
  Relational Operator1/1 -> NOT1/1, Gain1/1, Mux/3  "PWM_VH"
  Relational Operator/1 -> NOT/1, Scope2/2, Mux/1  "PWM_UH"
  Repeating Sequence/1 -> Compare To Constant/1, Scope/1, Relational Operator1/2, Scope2/3, Relational Operator/2, Relational Operator2/2  "PWM_Cnt"
  Relational Operator2/1 -> NOT2/1, Gain/1, Mux/5  "PWM_WH"
  NOT1/1 -> Mux/4
  NOT/1 -> Mux/2
  NOT2/1 -> Mux/6
  Mux/1 -> PWM/1
  In5/1 -> Scope/4, Relational Operator2/1  "Duty_W"
  Compare To Constant/1 -> Scope2/4, CaptureEna/1  "CaptureEna"
  Gain/1 -> Scope2/6  "PWM_WH"
  Gain1/1 -> Scope2/5  "PWM_VH"
  In1/1 -> Scope2/1, Relational Operator/1, Scope/2  "Duty_U"
  In3/1 -> Scope/3, Relational Operator1/1  "Duty_V"

== system MtrCtrl_24V/SpdCtrl ==
  SpdRef : Inport
  SpdFb : Inport  Port=2
  Sat : Inport  Port=3
  Tload : Inport  Port=4
  Add : Sum
  Gain : Gain  Gain=23
  Saturation : Saturate  UpperLimit=2000  LowerLimit=-2800
  Scope1 : Scope
  Scope5 : Scope  NumInputPorts=2
  Subsystem1 : Subsystem
  CurSet : Outport
  wires:
  Subsystem1/1(PIOut) -> Scope1/1, Add/1  "SpdPIOut"
  SpdFb/1 -> Subsystem1/2(Fbk), Scope5/2
  SpdRef/1 -> Saturation/1
  Gain/1 -> Add/2
  Sat/1 -> Subsystem1/3(Sat)
  Add/1 -> CurSet/1
  Tload/1 -> Gain/1
  Saturation/1 -> Scope5/1, Subsystem1/1(Ref)
